simulink model "robot_echant_etu"  (R2019a)
settings: Solver=VariableStepAuto  StartTime=0.0  StopTime=tf  RelTol=1e-3
values from neighbouring files (symbols this model uses):
  K = -place(A,B,poles)    [matrices.m]    (also in simu_robot_etu.m = [0.6700,19.9055,1.0747,1.9614])
  ue = 0    [simu_robot_etu.m]
  x0 = [0 pi/10 0 0]'    [simu_robot_etu.m]
  xe = [0 0 0 0]'    [simu_robot_etu.m]
undefined symbols (not defined in the file or in its folder): DiscIntNeverNeededParam
libraries: simulink x1
settings Model: Creator=nravalos  LastModifiedBy=mbenahme

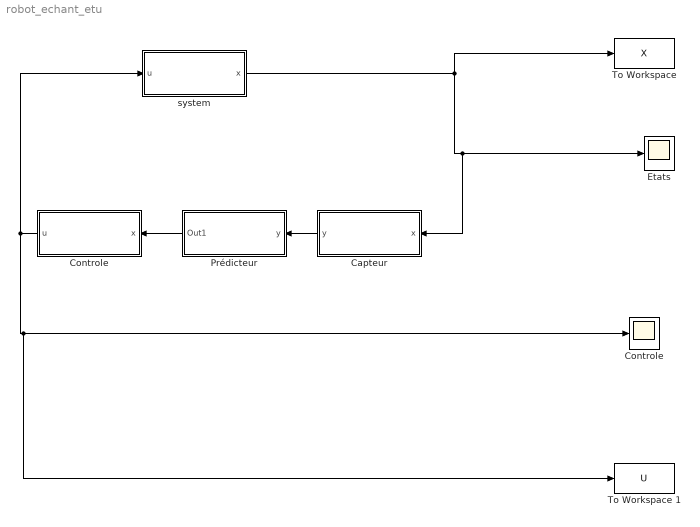
== system robot_echant_etu ==
  Capteur : Subsystem
  Controle : Subsystem
  "Controle " : Scope
  Etats : Scope
  Prédicteur : Subsystem
  "To Workspace " : ToWorkspace  VariableName=X  SaveFormat=Timeseries  SampleTime=-1
  "To Workspace 1 " : ToWorkspace  VariableName=U  SaveFormat=Timeseries  SampleTime=-1
  system : Subsystem
  wires:
  system/1(x) -> Capteur/1(x), Etats/1, "To Workspace "/1
  Controle/1(u) -> system/1("u "), "To Workspace 1 "/1, "Controle "/1
  Capteur/1(y) -> Prédicteur/1(y)
  Prédicteur/1(Out1) -> Controle/1(x)

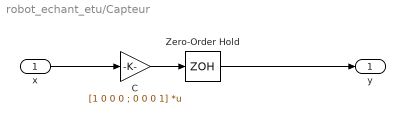
== system robot_echant_etu/Capteur ==
  x : Inport
  C : Gain  Gain=[1 0 0 0 ; 0 0 0 1]  Multiplication=Matrix(K*u)
  Zero-Order Hold : ZeroOrderHold  SampleTime=1e-3
  y : Outport
  wires:
  x/1 -> C/1
  C/1 -> Zero-Order Hold/1
  Zero-Order Hold/1 -> y/1

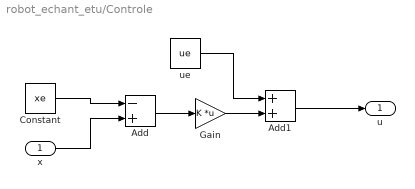
== system robot_echant_etu/Controle ==
  x : Inport
  Add : Sum  Inputs=-+
  Add1 : Sum
  Constant : Constant  Value=xe
  Gain : Gain  Gain=K  Multiplication=Matrix(K*u)
  ue : Constant  Value=ue
  u : Outport
  wires:
  x/1 -> Add/2
  Add1/1 -> u/1
  ue/1 -> Add1/1
  Gain/1 -> Add1/2
  Constant/1 -> Add/1
  Add/1 -> Gain/1

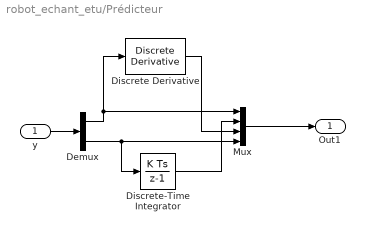
== system robot_echant_etu/Prédicteur ==
  y : Inport
  Demux : Demux  Outputs=2
  Discrete Derivative : simulink/Discrete/Discrete Derivative  gainval=1.0  ICPrevScaledInput=0.0  OutMin=[]  OutMax=[]  OutDataType=fixdt(1, 16)  OutScaling=2^-10  DoSatur=off
  Discrete-Time Integrator : DiscreteIntegrator  SampleTime=1e-3  ICPrevOutput=DiscIntNeverNeededParam  ICPrevScaledInput=DiscIntNeverNeededParam
  Mux : Mux
  Out1 : Outport
  wires:
  y/1 -> Demux/1
  Demux/1 -> Discrete Derivative/1, Mux/1
  Demux/2 -> Discrete-Time Integrator/1, Mux/4
  Mux/1 -> Out1/1
  Discrete Derivative/1 -> Mux/3
  Discrete-Time Integrator/1 -> Mux/2

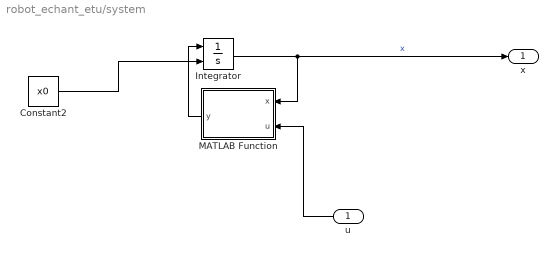
== system robot_echant_etu/system ==
  "u " : Inport
  Constant2 : Constant  Value=x0
  Integrator : Integrator  InitialConditionSource=external
  MATLAB Function : MATLAB Function  TreatAsAtomicUnit=on
  x : Outport
  wires:
  "u "/1 -> MATLAB Function/2(u)
  Integrator/1 -> x/1, MATLAB Function/1(x)  "x"
  MATLAB Function/1(y) -> Integrator/1
  Constant2/1 -> Integrator/2

== matlab function robot_echant_etu/system/MATLAB Function ==
  data: x input; u input; y output
function y = fcn(x, u)

y = fonction(x,u);
